simulink model "n"  (R2020a)
settings: Solver=VariableStepAuto  StartTime=0.0  StopTime=10
undefined symbols (not defined in the file or in its folder): k
settings Model: Creator=Mostafa Mahmoud  LastModifiedBy=Mostafa Mahmoud
settings DataIOCC: SaveState=on  ReturnWorkspaceOutputs=off
settings DebuggingCC: ArithmeticOperatorsInVariantConditions=warning
settings SFSimCC: CustomCodeUndefinedFunction=UseInterfaceOnly

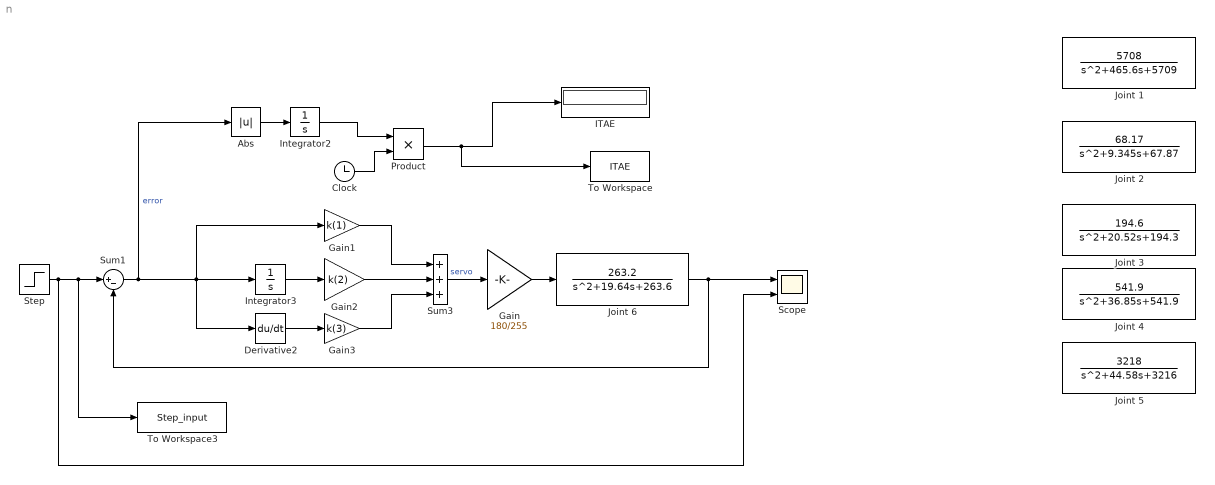
== system n ==
  Abs : Abs
  Clock : Clock
  Derivative2 : Derivative
  Gain : Gain  Gain=180/255
  Gain1 : Gain  Gain=k(1)
  Gain2 : Gain  Gain=k(2)
  Gain3 : Gain  Gain=k(3)
  ITAE : Display
  Integrator2 : Integrator
  Integrator3 : Integrator
  Joint 1 : TransferFcn  Numerator=[5708]  Denominator=[1 465.6 5709]
  Joint 2 : TransferFcn  Numerator=[68.17]  Denominator=[1 9.345 67.87]
  Joint 3 : TransferFcn  Numerator=[194.6]  Denominator=[1 20.52 194.3]
  Joint 4 : TransferFcn  Numerator=[541.9]  Denominator=[1 36.85 541.9]
  Joint 5 : TransferFcn  Numerator=[3218]  Denominator=[1 44.58 3216]
  Joint 6 : TransferFcn  Numerator=[263.2]  Denominator=[1 19.64 263.6]
  Product : Product
  Scope : Scope  NumInputPorts=2
  Step : Step  SampleTime=0
  Sum1 : Sum  Inputs=|+-
  Sum3 : Sum  Inputs=+++
  To Workspace : ToWorkspace  VariableName=ITAE  SampleTime=-1
  To Workspace3 : ToWorkspace  VariableName=Step_input  SampleTime=-1
      settings: Save2DSignal=2-D array (concatenate along first dimension)
  wires:
  Abs/1 -> Integrator2/1
  Integrator2/1 -> Product/1
  Clock/1 -> Product/2
  Product/1 -> To Workspace/1, ITAE/1
  Gain3/1 -> Sum3/3
  Derivative2/1 -> Gain3/1
  Gain2/1 -> Sum3/2
  Integrator3/1 -> Gain2/1
  Gain1/1 -> Sum3/1
  Sum1/1 -> Abs/1, Gain1/1, Derivative2/1, Integrator3/1  "error"
  Sum3/1 -> Gain/1  "servo"
  Step/1 -> Scope/2, To Workspace3/1, Sum1/1
  Gain/1 -> Joint 6/1
  Joint 6/1 -> Scope/1, Sum1/2
